simulink model "VerificaLQG_27042026"  (R2025b)
settings: Solver=VariableStepAuto  StartTime=0.0  StopTime=20.0  RelTol=1e-3
values from neighbouring files (symbols this model uses):
  A = double(subs(A_sym, [x; u], [x_star; u_star]))    [Esame_27042026.m]
  B = double(subs(B_sym, [x; u], [x_star; u_star]))    [Esame_27042026.m]
  C = eye(n)    [Esame_27042026.m]
  D = zeros(n, m)    [Esame_27042026.m]
  K_LQR_i = K_LQR(:, n+1:end)    [Esame_27042026.m]
  K_LQR_x = K_LQR(:, 1:n)    [Esame_27042026.m]
undefined symbols (not defined in the file or in its folder): A_kf, B_kf, C_kf, C_LQG, Q_cov, R_cov, x0_LQR, xref_LQG
libraries: simulink x2
settings Model: Creator=inggi  LastModifiedBy=salvo

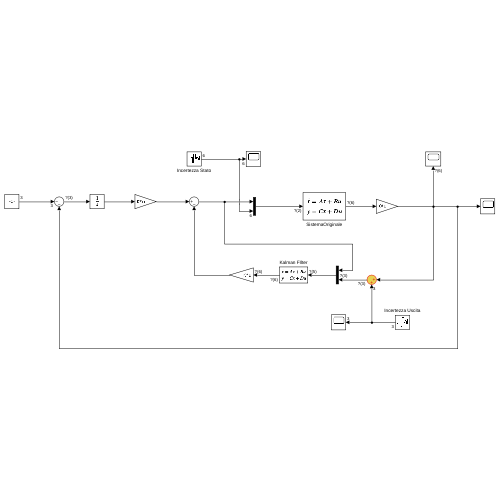
[thumbnail: Simulink's stored preview of the top-level diagram]
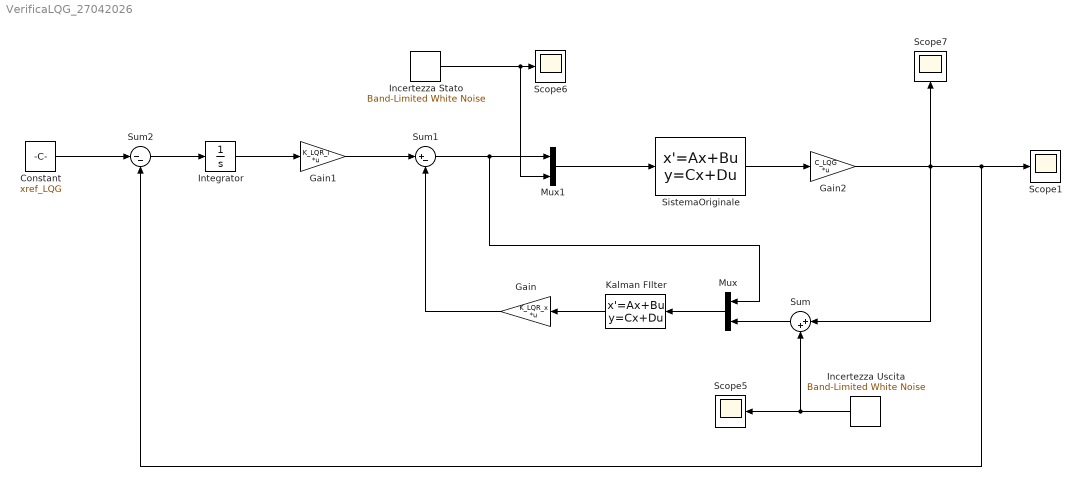
== system VerificaLQG_27042026 ==
  Constant : Constant  Value=xref_LQG
  Gain : Gain  Gain=K_LQR_x  Multiplication=Matrix(K*u)
  Gain1 : Gain  Gain=K_LQR_i  Multiplication=Matrix(K*u)
  Gain2 : Gain  Gain=C_LQG  Multiplication=Matrix(K*u)
  Incertezza Stato : simulink/Sources/Band-Limited White Noise  Cov=diag(Q_cov)  Ts=0.1  seed=[23341]
  Incertezza Uscita : simulink/Sources/Band-Limited White Noise  Cov=diag(R_cov)  Ts=0.1  seed=[23341]
  Integrator : Integrator
  Kalman FIlter : StateSpace  A=A_kf  B=B_kf  C=C_kf  D=zeros(6,5)  InitialCondition=0
  Mux : Mux  Inputs=2
  Mux1 : Mux  Inputs=2
  Scope{1,5..7} (4 alike) : Scope
      Scope5 settings: DataLoggingVariableName=ScopeData5
      Scope6 settings: ActiveDisplayYMinimum=-76.650319692534367  ActiveDisplayYMaximum=39.186003026903144  DataLoggingVariableName=ScopeData6
      Scope7 settings: DataLoggingVariableName=ScopeData7
  SistemaOriginale : StateSpace  A=A  B=B  C=C  D=D  InitialCondition=x0_LQR
  Sum : Sum  Inputs=|++
  Sum1 : Sum  Inputs=|+-
  Sum2 : Sum  Inputs=|--
  wires:
  Incertezza Uscita/1 -> Sum/2, Scope5/1
  Mux/1 -> Kalman FIlter/1
  Sum/1 -> Mux/2
  Mux1/1 -> SistemaOriginale/1
  Incertezza Stato/1 -> Mux1/2, Scope6/1
  Kalman FIlter/1 -> Gain/1
  Sum1/1 -> Mux/1, Mux1/1
  Gain/1 -> Sum1/2
  Gain1/1 -> Sum1/1
  Integrator/1 -> Gain1/1
  Sum2/1 -> Integrator/1
  Constant/1 -> Sum2/1
  SistemaOriginale/1 -> Gain2/1
  Gain2/1 -> Sum/1, Scope7/1, Scope1/1, Sum2/2
